simulink model "MotorGenerator2Basic_test_harness"  (R2020b)
settings: Solver=VariableStepAuto  StartTime=0.0  StopTime=t_end  RelTol=1e-3  AbsTol=1e-3
PreLoadFcn:
  | MotorGenerator2Basic_setup
undefined symbols (not defined in the file or in its folder): testharness
libraries: nesl_utility x2, fl_lib x1, EVComponents_utility_lib x1
settings Model: Creator=isaacito  LastModifiedBy=isaacito
settings SolverCC: AutoScaleAbsTol=off
settings DebuggingCC: SymbolicDimsDataTypeCodeGenerationDiagnostic=none
settings SFSimCC: CustomCodeUndefinedFunction=UseInterfaceOnly
settings SimscapeCC: SimscapeLogType=all  SimscapeLogSimulationStatistics=on  SimscapeLogLimitData=off  SimscapeLogDataHistory=10000

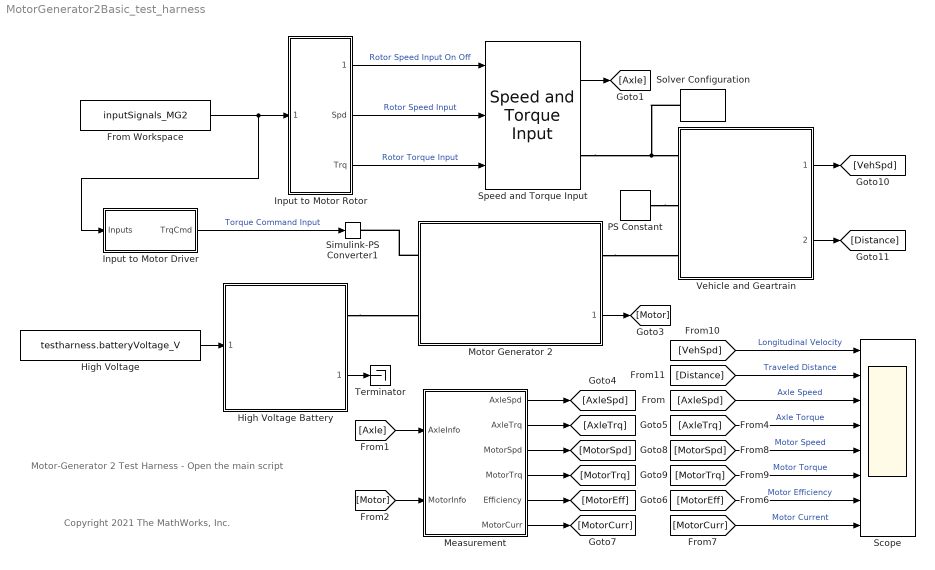
== system MotorGenerator2Basic_test_harness ==
  note: Copyright 2021 The MathWorks, Inc.
  note: Motor-Generator 2 Test Harness
      | - Open the main script
  From Workspace : FromWorkspace  VariableName=inputSignals_MG2  OutDataTypeStr=Bus: inputBus_MG2  Interpolate=off  OutputAfterFinalValue=Holding final value
      settings: AttributesFormatString=%<OutDataTypeStr>
  High Voltage : Constant  Value=testharness.batteryVoltage_V
  High Voltage Battery : Subsystem  ReferencedSubsystem=BatteryForTest_refsub
      settings: PortSchema="{\"entries\":[{\"content\":{\"sides\":[{\"content\":{\"connectorIds\":[\"In1\"]},\"type\":\"ConnectorPlacement.EquallySpacedRectSide\",\"uuid\":\"6ec42dc2-af13-403d-bb44-bbfe17049ebb\"},{\"content\":{\"connectorIds\":[\"RConn1\",\"Out1\"],\"side\":\"RIGHT\"},\"type\":\"ConnectorPlacement.EquallySpacedRectSide\",\"uuid\":\"18b43a22-b216-415c-b9ff-5dd426481655\"},{\"content\":{\"connectorIds\":[],\"side\":\"TOP\"},\"type\":\"ConnectorPlacement.EquallySpacedRectSide\",\"uuid\":\"9ddf6635-2c27-427a-8c83-df626a0e9ed3\"},{\"content\":{\"connectorIds\":[],\"side\":\"HIDDEN\"},\"type\":\"ConnectorPlacement.EquallySpacedRectSide\",\"uuid\":\"332981be-c8a8-46f3-86be-153015cc7779\"}]},\"type\":\"ConnectorPlacement.EquallySpacedConnector\",\"uuid\":\"0a64d723-305c-452f-a915-e14881ea19f7\"}],\"packageUris\":[\"http://schema.mathworks.com/mf0/Connector/R2020b\"],\"version\":\"1.0\"}"
  Input to Motor Driver : Subsystem
  Input to Motor Rotor : Subsystem
  Measurement : Subsystem
  Motor Generator 2 : Subsystem  ReferencedSubsystem=MotorGenerator2Basic_refsub
      settings: PortSchema="{\"entries\":[{\"content\":{\"sides\":[{\"content\":{\"connectorIds\":[\"LConn2\",\"LConn1\"]},\"type\":\"ConnectorPlacement.EquallySpacedRectSide\",\"uuid\":\"9065e87b-4b12-4906-a348-add511aef997\"},{\"content\":{\"connectorIds\":[\"RConn1\",\"Out1\"],\"side\":\"RIGHT\"},\"type\":\"ConnectorPlacement.EquallySpacedRectSide\",\"uuid\":\"505b00e5-dae1-4af4-957c-e679e57e315e\"},{\"content\":{\"connectorIds\":[],\"side\":\"TOP\"},\"type\":\"ConnectorPlacement.EquallySpacedRectSide\",\"uuid\":\"1548ce11-ff15-4884-816d-b086c6e11573\"},{\"content\":{\"connectorIds\":[],\"side\":\"HIDDEN\"},\"type\":\"ConnectorPlacement.EquallySpacedRectSide\",\"uuid\":\"3ffc3eea-1039-4ad2-84c6-cfb13bcd9ba2\"}]},\"type\":\"ConnectorPlacement.EquallySpacedConnector\",\"uuid\":\"a56170af-522a-47ae-83fe-bc261b41ce3e\"}],\"packageUris\":[\"http://schema.mathworks.com/mf0/Connector/R2020b\"],\"version\":\"1.0\"}"
  PS Constant : fl_lib/Physical Signals/Sources/PS Constant  constant=0 N
      settings: AttributesFormatString=%<constant>
  Scope : Scope  NumInputPorts=8
  Simulink-PS Converter1 : nesl_utility/Simulink-PS Converter  PhysicalDomain=network_engine_domain  SubClassName=ps_input  LeftPortType=input  RightPortType=output  PseudoPeriodic=off  Frequencies=[]  NoiseDistribution=none  NoiseParameters=[]  Unit=N*m  AffineConversion=off  FilteringAndDerivatives=provide  SimscapeFilterOrder=1  InputFilterTimeConstant=0.001  UdotUserProvided=0
      settings: SourceProductName=Utilities
  Solver Configuration : nesl_utility/Solver Configuration  PhysicalDomain=network_engine_domain  SubClassName=solver  LeftPortType=input  RightPortType=generic  Tones=[]  Harmonics=[]  SimulateNoise=off  Profile=off  UseLocalSampling=off  EnableSwitchedLinearOptims=on  FrequencyDomain=off  UseCCode=off  RelTol=0.001  AbsTol=1e-06  MinStep=1e-09  ToWorkspace=off  RevertToSquareIcSolve=off  NumHomotopyIterations=100  PhasorMode=off  PhasorModeNumHarmonics=1  DoDC=off  ResidualTolerance=1e-09  UseLocalSolver=off  LocalSolverChoice=NE_BACKWARD_EULER_ADVANCER  LocalSolverSampleTime=0.001  DoFixedCost=off  MaxNonlinIter=3  MaxModeIter=2  ComputeImpulses=off  ImpulseIterations=2  LinearAlgebra=auto  EquationFormulation=NE_TIME_EF  DelaysMemoryBudget=1024  AutomaticFiltering=on  FilteringTimeConstant=0.001  PartitionStorageMethod=AS_NEEDED  PartitionMemoryBudget=1024  PartitionMethod=ROBUST
      settings: SourceProductName=Utilities
  Speed and Torque Input : EVComponents_utility_lib/Speed and Torque Input  t_friction=10000  t_locked=10000  w_tol=0.001  initial_state_locked=sdl.enum.initial_lock.unlocked
  Terminator : Terminator
  Vehicle and Geartrain : Subsystem  ReferencedSubsystem=VehicleForTest_refsub
      settings: PortSchema="{\"entries\":[{\"content\":{\"sides\":[{\"content\":{\"connectorIds\":[\"LConn1\",\"LConn3\",\"LConn2\"]},\"type\":\"ConnectorPlacement.EquallySpacedRectSide\",\"uuid\":\"c975ecd5-3624-4c19-9a80-acedd8bc41a3\"},{\"content\":{\"connectorIds\":[\"Out1\",\"Out2\"],\"side\":\"RIGHT\"},\"type\":\"ConnectorPlacement.EquallySpacedRectSide\",\"uuid\":\"910143c3-3967-4448-a629-d08cf6777789\"},{\"content\":{\"connectorIds\":[],\"side\":\"TOP\"},\"type\":\"ConnectorPlacement.EquallySpacedRectSide\",\"uuid\":\"7a417a30-364f-4b70-8ba2-82e05b7f8ad5\"},{\"content\":{\"connectorIds\":[],\"side\":\"HIDDEN\"},\"type\":\"ConnectorPlacement.EquallySpacedRectSide\",\"uuid\":\"66b5b01a-20fa-4f6a-8c11-38a64c540bf5\"}]},\"type\":\"ConnectorPlacement.EquallySpacedConnector\",\"uuid\":\"d97c4709-181f-4fdd-bd6d-fe96f1a8d0ed\"}],\"packageUris\":[\"http://schema.mathworks.com/mf0/Connector/R2020b\"],\"version\":\"1.0\"}"
  wires:
  High Voltage/1 -> High Voltage Battery/1
  Motor Generator 2/1 -> [Motor]
  From Workspace/1 -> Input to Motor Driver/1(Inputs), Input to Motor Rotor/1(Inputs)
  Input to Motor Rotor/3(Trq) -> Speed and Torque Input/3  "Rotor Torque Input"
  Speed and Torque Input/1 -> [Axle]
  Input to Motor Rotor/2(Spd) -> Speed and Torque Input/2  "Rotor Speed Input"
  Input to Motor Rotor/1(Spd_OnOff) -> Speed and Torque Input/1  "Rotor Speed Input On Off"
  Input to Motor Driver/1(TrqCmd) -> Simulink-PS Converter1/1  "Torque Command Input"
  [Axle] -> Measurement/1(AxleInfo)
  [Motor] -> Measurement/2(MotorInfo)
  Measurement/1(AxleSpd) -> [AxleSpd]
  Measurement/2(AxleTrq) -> [AxleTrq]
  Measurement/5(Efficiency) -> [MotorEff]
  Measurement/6(MotorCurr) -> [MotorCurr]
  Measurement/3(MotorSpd) -> [MotorSpd]
  Measurement/4(MotorTrq) -> [MotorTrq]
  [VehSpd] -> Scope/1  "Longitudinal Velocity"
  [Distance] -> Scope/2  "Traveled Distance"
  [AxleSpd] -> Scope/3  "Axle Speed"
  [AxleTrq] -> Scope/4  "Axle Torque"
  [MotorSpd] -> Scope/5  "Motor Speed"
  [MotorTrq] -> Scope/6  "Motor Torque"
  [MotorEff] -> Scope/7  "Motor Efficiency"
  [MotorCurr] -> Scope/8  "Motor Current"
  Vehicle and Geartrain/1 -> [VehSpd]
  Vehicle and Geartrain/2 -> [Distance]
  High Voltage Battery/1 -> Terminator/1
  connections:
  High Voltage Battery/RConn1 -- Motor Generator 2/LConn1
  Motor Generator 2/LConn2 -- Simulink-PS Converter1/RConn1
  Speed and Torque Input/RConn1 -- Solver Configuration/RConn1 -- Vehicle and Geartrain/LConn1
  Motor Generator 2/RConn1 -- Vehicle and Geartrain/LConn2
  PS Constant/RConn1 -- Vehicle and Geartrain/LConn3

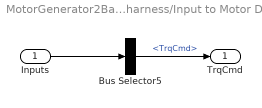
== system MotorGenerator2Basic_test_harness/Input to Motor Driver ==
  Inputs : Inport
  Bus Selector5 : BusSelector  OutputSignals=TrqCmd
  TrqCmd : Outport
  wires:
  Bus Selector5/1 -> TrqCmd/1  "<TrqCmd>"
  Inputs/1 -> Bus Selector5/1

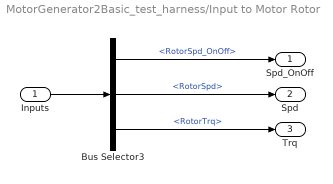
== system MotorGenerator2Basic_test_harness/Input to Motor Rotor ==
  Inputs : Inport
  Bus Selector3 : BusSelector  OutputSignals=RotorSpd_OnOff,RotorSpd,RotorTrq
  Spd_OnOff : Outport
  Spd : Outport  Port=2
  Trq : Outport  Port=3
  wires:
  Bus Selector3/2 -> Spd/1  "<RotorSpd>"
  Inputs/1 -> Bus Selector3/1
  Bus Selector3/1 -> Spd_OnOff/1  "<RotorSpd_OnOff>"
  Bus Selector3/3 -> Trq/1  "<RotorTrq>"

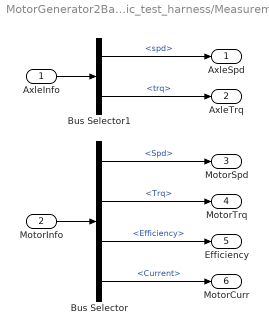
== system MotorGenerator2Basic_test_harness/Measurement ==
  AxleInfo : Inport
  MotorInfo : Inport  Port=2
  Bus Selector : BusSelector  OutputSignals=Spd,Trq,Efficiency,Current
  Bus Selector1 : BusSelector  OutputSignals=spd,trq
  AxleSpd : Outport
  AxleTrq : Outport  Port=2
  MotorSpd : Outport  Port=3
  MotorTrq : Outport  Port=4
  Efficiency : Outport  Port=5
  MotorCurr : Outport  Port=6
  wires:
  AxleInfo/1 -> Bus Selector1/1
  Bus Selector1/1 -> AxleSpd/1  "<spd>"
  Bus Selector1/2 -> AxleTrq/1  "<trq>"
  MotorInfo/1 -> Bus Selector/1
  Bus Selector/1 -> MotorSpd/1  "<Spd>"
  Bus Selector/2 -> MotorTrq/1  "<Trq>"
  Bus Selector/4 -> MotorCurr/1  "<Current>"
  Bus Selector/3 -> Efficiency/1  "<Efficiency>"
